simulink model "Ideal_CPS_F_as_zero"  (R2022b)
settings: Solver=VariableStepAuto  StartTime=0.0  StopTime=10.0  RelTol=1e-3
values from neighbouring files (symbols this model uses):
  c = 2*dampratio*sqrt(k*M)    [CPS_sims_and_analysis.m]    (also in command_limits_check.m; ringdown-circcyl-M10-d0_001-F1-workspace.mat = 0.125663706144; setup_CPS_parameters.m)
  k = (2*pi*f_nat)^2*M    (= 394.784176044)    [CPS_sims_and_analysis.m]    (also in command_limits_check.m = 98.6960440109; ringdown-circcyl-M10-d0_001-F1-workspace.mat; setup_CPS_parameters.m = 98.6960440109)
  M = 10    [CPS_sims_and_analysis.m]    (also in command_limits_check.m; ringdown-circcyl-M10-d0_001-F1-workspace.mat; setup_CPS_parameters.m)
  start_position_cm = 10    [command_limits_check.m]    (also in ringdown-circcyl-M10-d0_001-F1-workspace.mat = 0.0117475; setup_CPS_parameters.m = 0)
  T = 0.0002    [ringdown-circcyl-M10-d0_001-F1-workspace.mat]    (also in setup_CPS_parameters.m = 0.001)
undefined symbols (not defined in the file or in its folder): DiscIntNeverNeededParam
settings Model: Creator=eericks1  LastModifiedBy=eericks1
settings DataIOCC: ReturnWorkspaceOutputs=off

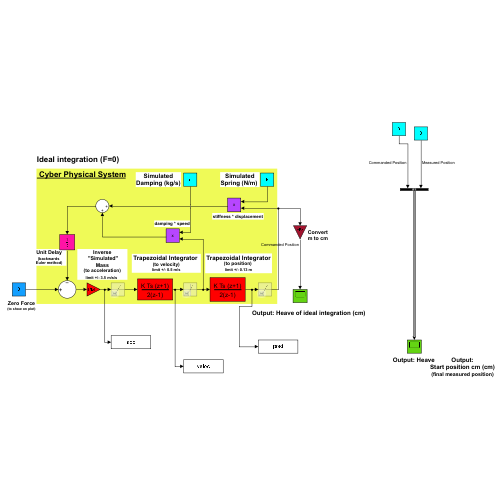
[thumbnail: Simulink's stored preview of the top-level diagram]
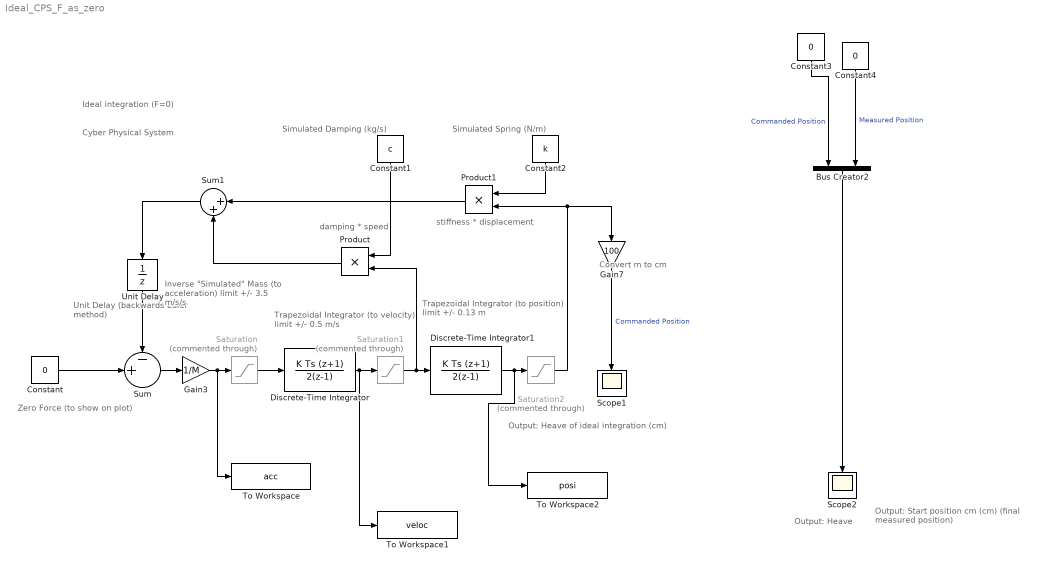
== system Ideal_CPS_F_as_zero ==
  note: Cyber Physical System
  note: stiffness * displacement
  note: Simulated
      | Spring (N/m)
  note: Trapezoidal Integrator
      | (to position)
      | limit +/- 0.13 m
  note: Simulated
      | Damping (kg/s)
  note: Unit Delay
      | (backwards
      | Euler method)
  note: Inverse
      | "Simulated"
      | Mass
      | (to acceleration)
      | limit +/- 3.5 m/s/s
  note: Trapezoidal Integrator
      | (to velocity)
      | limit +/- 0.5 m/s
  note: damping * speed
  note: Ideal integration (F=0)
  note: Zero Force
      | (to show on plot)
  note: Output: Heave of ideal integration (cm)
  note: Convert
      | m to cm
  note: Output: Heave
  note: Output:
      | Start position cm (cm)
      | (final measured position)
  Bus Creator2 : BusCreator  Inputs=2
  Constant : Constant  Value=0  SampleTime=T
  Constant1 : Constant  Value=c  SampleTime=T
  Constant2 : Constant  Value=k  SampleTime=T
  Constant3 : Constant  Value=0  SampleTime=T
  Constant4 : Constant  Value=0  SampleTime=T
  Discrete-Time Integrator : DiscreteIntegrator  IntegratorMethod=Integration: Trapezoidal  SampleTime=-1  UpperSaturationLimit=0.5  LowerSaturationLimit=-0.5  ICPrevOutput=DiscIntNeverNeededParam  ICPrevScaledInput=DiscIntNeverNeededParam
  Discrete-Time Integrator1 : DiscreteIntegrator  IntegratorMethod=Integration: Trapezoidal  InitialCondition=start_position_cm/100  SampleTime=-1  UpperSaturationLimit=.13  LowerSaturationLimit=-.13  ICPrevOutput=DiscIntNeverNeededParam  ICPrevScaledInput=DiscIntNeverNeededParam
  Gain3 : Gain  Gain=1/M
  Gain7 : Gain  Gain=100
  Product : Product
  Product1 : Product
  Saturation : Saturate  Commented=through  UpperLimit=3.5  LowerLimit=-3.5
  Saturation1 : Saturate  Commented=through
  Saturation2 : Saturate  Commented=through  UpperLimit=0.13  LowerLimit=-0.13
  Scope1 : Scope
  Scope2 : Scope
  Sum : Sum  Inputs=-+|
  Sum1 : Sum  Inputs=|++
  To Workspace : ToWorkspace  VariableName=acc  SampleTime=-1
  To Workspace1 : ToWorkspace  VariableName=veloc  SampleTime=-1
  To Workspace2 : ToWorkspace  VariableName=posi  SampleTime=-1
  Unit Delay : UnitDelay  InitialCondition=start_position_cm*k/100  SampleTime=-1  HasFrameUpgradeWarning=on
  wires:
  Saturation/1 -> Discrete-Time Integrator/1
  Saturation1/1 -> Product/2, Discrete-Time Integrator1/1
  Product1/1 -> Sum1/1
  Discrete-Time Integrator1/1 -> To Workspace2/1, Saturation2/1
  Constant2/1 -> Product1/1
  Saturation2/1 -> Gain7/1, Product1/2
  Product/1 -> Sum1/2
  Discrete-Time Integrator/1 -> To Workspace1/1, Saturation1/1
  Constant1/1 -> Product/1
  Unit Delay/1 -> Sum/1
  Sum/1 -> Gain3/1
  Gain3/1 -> To Workspace/1, Saturation/1
  Sum1/1 -> Unit Delay/1
  Constant/1 -> Sum/2
  Gain7/1 -> Scope1/1  "Commanded Position"
  Constant3/1 -> Bus Creator2/1  "Commanded Position"
  Constant4/1 -> Bus Creator2/2  "Measured Position"
  Bus Creator2/1 -> Scope2/1
